simulink model "DeePC_SimulinkV4"  (R2025b)
settings: Solver=FixedStepDiscrete  StartTime=0.0  StopTime=12  FixedStep=0.001  RelTol=1e-3  EnableMultiTasking=on
PreLoadFcn:
  | if ~exist('Ts', 'var')
  | Ts = 0.001;
  | end
  | if ~exist('FPGA_Frequency', 'var')
  | FPGA_Frequency = 75000000;
  | end
  | if ~exist('Tpwm', 'var')
  | Tpwm = 0.005;
  | end
model workspace (MAT data in the model file):
  Sig = Simulink.Signal
  Sig.Dimensions = -1
  Sig.DimensionsMode = 'auto'
  Sig.Complexity = 'auto'
  Sig.SampleTime = -1
  Sig.SamplingMode = 'auto'
  Sig.DataType = 'auto'
values from neighbouring files (symbols this model uses):
  f_pre_r = makeParam(DataStruct.f)    [ExperimentControlCenter_V3.m]
  H = makeParam(DataStruct.H)    [ExperimentControlCenter_V3.m]
  H_p = makeParam(DataStruct.H_p)    [ExperimentControlCenter_V3.m]
  IOscale = makeParam(DataStruct.IOscale)    [ExperimentControlCenter_V3.m]
  l = makeParam(l_val)    [ExperimentControlCenter_V3.m]
  lambda_g = makeParam(lambda_g_list(1))    [ExperimentControlCenter_V3.m]
  lambda_y = 5e2    (= 500)    [ExperimentControlCenter_V3.m]
  N = makeParam(DataStruct.N)    [ExperimentControlCenter_V3.m]
  T_ini = makeParam(DataStruct.T_ini)    [ExperimentControlCenter_V3.m]
  T_switch = makeParam(T_switch_val)    [ExperimentControlCenter_V3.m]
  Ts_ctrl_sl = makeParam(Ts_ctrl)    [ExperimentControlCenter_V3.m]
  U_f = makeParam(DataStruct.U_f)    [ExperimentControlCenter_V3.m]
  Y_f = makeParam(DataStruct.Y_f)    [ExperimentControlCenter_V3.m]
undefined symbols (not defined in the file or in its folder): DiscIntNeverNeededParam, IO397, Pull, pull, up
libraries: simulink x6, speedgoatlib_fpga_analog_io x3, speedgoatlib_fpga_quadrature x3, speedgoatlib_fpga_dio x1, speedgoatlib_fpga_inta x1, speedgoatlib_interrupt x1, speedgoatlib_fpga_pwm x1, speedgoatlib_fpga x1
settings Model: SimulationMode=external  ExtModeEnableFloating=off  Creator=jeffrey.gruenig  LastModifiedBy=gertv
settings SolverCC: ConcurrentTasks=on  PositivePriorityOrder=on  AutoInsertRateTranBlk=on
settings DataIOCC: SaveFormat=StructureWithTime  SaveOutput=off  SaveTime=off
settings OptimizationCC: BlockReduction=off  DefaultParameterBehavior=Inlined  OptimizeBlockIOStorage=off  EnhancedBackFolding=on  PassReuseOutputArgsThreshold=0.0  OptimizeBlockOrder=speed  DifferentSizesBufferReuse=on
settings DebuggingCC: UnderspecifiedInitializationDetection=Classic  MergeDetectMultiDrivingBlocksExec=none  TasksWithSamePriorityMsg=none  ParameterTunabilityLossMsg=error  AllowSymbolicDim=off
settings HardwareCC: ProdBitPerLong=64.0  ProdLongLongMode=on  ProdHWDeviceType=Intel->x86-64 (Linux 64)
settings ModelReferenceCC: PropagateSignalLabelsOutOfModel=off
settings RTWCC: SystemTargetFile=speedgoat.tlc  TLCOptions=-p0  TemplateMakefile=slrealtime_default_tmf  GenerateReport=on  RTWVerbose=off  Toolchain=Simulink Real-Time Toolchain  LaunchReport=on  CodeExecutionProfiling=on  TargetLang=C++  Description=Speedgoat Real-Time Target Machine
settings CodeAppCC: ForceParamTrailComments=on  OperatorAnnotations=on
settings SimulinkRealTimeTargetCC: SLRTFileLogMaxRuns=1.0  ExtModeMaxTrigDuration=10.0  ExtModeStaticAllocSize=1000000.0  ExtModeTransport=0.0  MultiwordLength=2048.0  DynamicStringBufferSize=256.0  PreserveMATLABNamespacesInGeneratedCode=on  SubcomponentCodeInterfacePackaging=Reusable function  InstructionSetFMA=off  LogToMDFFile=off

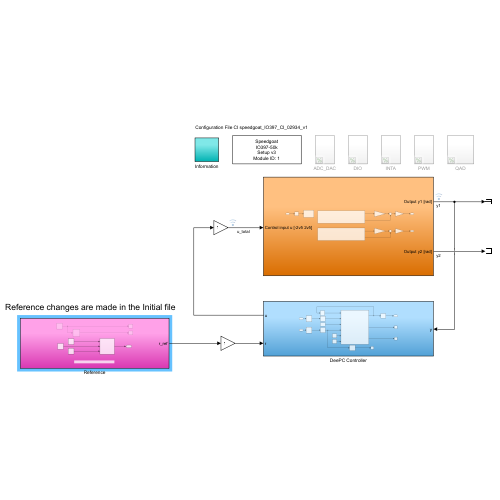
[thumbnail: Simulink's stored preview of the top-level diagram]
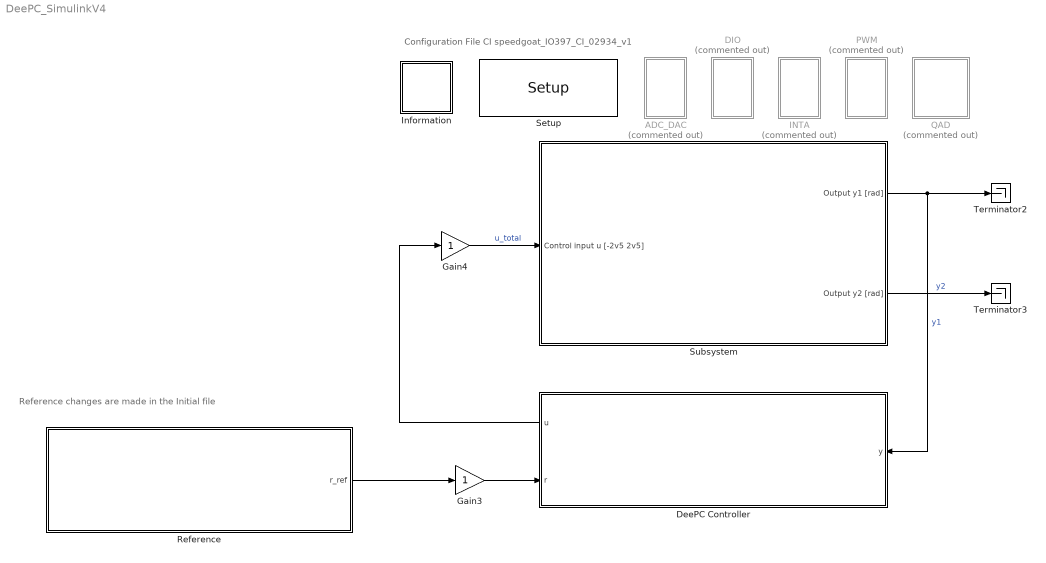
== system DeePC_SimulinkV4 ==
  note: Reference changes are made in the Initial file
  note: Configuration File CI speedgoat_IO397_CI_02934_v1
  ADC_DAC : Subsystem  Commented=on
  DIO : Subsystem  Commented=on
  DeePC Controller : Subsystem
      settings: PortSchema="{\"entries\":[{\"content\":{\"sides\":[{\"content\":{\"connectorIds\":[\"In1\"]},\"type\":\"ConnectorPlacement.EquallySpacedRectSide\",\"uuid\":\"2e71bc44-88de-4f6b-852e-26b86c3fb698\"},{\"content\":{\"connectorIds\":[\"Out1\",\"In2\"],\"side\":\"RIGHT\"},\"type\":\"ConnectorPlacement.EquallySpacedRectSide\",\"uuid\":\"c8a8557f-0bf5-47f4-bae2-a177ab114f93\"},{\"content\":{\"side\":\"TOP\"},\"type\":\"ConnectorPlacement.EquallySpacedRectSide\",\"uuid\":\"9add04b7-c795-4733-b5be-0ba9d1775d75\"},{\"content\":{\"side\":\"BOTTOM\"},\"type\":\"ConnectorPlacement.EquallySpacedRectSide\",\"uuid\":\"f8ea6dec-d938-4893-9b5d-ff6cf4332b98\"}]},\"type\":\"ConnectorPlacement.EquallySpacedConnector\",\"uuid\":\"ed5613c3-599d-4249-97c1-c6090c1efcc5\"}],\"packageUris\":[\"http://schema.mathworks.com/mf0/Connector/R2020b\"],\"version\":\"1.0\"}"
  Gain3 : Gain
  Gain4 : Gain
  INTA : Subsystem  Commented=on
  Information : Subsystem
  PWM : Subsystem  Commented=on
  QAD : Subsystem  Commented=on
  Reference : Subsystem
  Setup : speedgoatlib_fpga/Setup/Setup  board=IO397-50k  id=1  pciSlot=-1  device_id=1  bitstreamFilePath=C:\Users\gertv\Documents\Werk\Continuing Thesis\Matlab\GithubFolder\Section 9 - Experimental Results\ExperimentSet_up\DeePC_Exp  bitstreamFile=speedgoat_IO397_CI_02934_v1.mat  fpgaFreq=75000000  enableDma=off  rearEnb_1=off  rearIO_1=None  rearEnb_2=off  rearIO_2=None  ProgSpiFlash=off  ProgBPIFlash=off  useFpgaDmaController=off  dmaStopOnOverload=on  dmaModeSequential=on  dmaModeParallel=off  dmaTrigFixTime=on  dmaTrigA2B=off  dmaTriggerSourceSel=0  PullRPort15=pull-up 3.3V  PullRPort31=pull-up 3.3V  PullRPort47=pull-up 3.3V  PullRPort63=pull-up 3.3V  diffLineTermination_1=on  diffLineTermination_2=on  diffLineTermination_3=on  diffLineTermination_4=on  diffLineTermination_5=on  diffLineTermination_6=on  diffLineTermination_7=on  diffLineTermination_8=on  diffLineTermination_9=on  diffLineTermination_10=on  diffLineTermination_11=on  diffLineTermination_12=on  diffLineTermination_13=on  diffLineTermination_14=on  diffLineTermination_15=on  diffLineTermination_16=on  diffLineTermination_17=on  diffLineTermination_18=on  diffLineTermination_19=on  diffLineTermination_20=on  diffLineTermination_21=on  diffLineTermination_22=on  diffLineTermination_23=on  diffLineTermination_24=on  diffLineTermination_25=on  diffLineTermination_26=on  diffLineTermination_27=on  diffLineTermination_28=on  diffLineTermination_29=on  diffLineTermination_30=on  diffLineTermination_31=on  diffLineTermination_32=on  ioVoltageDropDown1=3.3V  pullResistorDropDown1_1=Pull-up  pullResistorDropDown1_2=Pull-up  pullResistorDropDown1_3=Pull-up  pullResistorDropDown1_4=Pull-up  pullResistorDropDown1_5=Pull-up  pullResistorDropDown1_6=Pull-up  pullResistorDropDown1_7=Pull-up  pullResistorDropDown1_8=Pull-up  ttlIsImplementedCheckBox1=off  pullResistorDropDown2=Pull-up  ioVoltageDropDown2=3.3V  ttlIsImplementedCheckBox2=off  pullResistorDropDown3=Pull-up  ioVoltageDropDown3=3.3V  ttlIsImplementedCheckBox3=off  pullResistorDropDown4=Pull-up  ioVoltageDropDown4=3.3V  ttlIsImplementedCheckBox4=off  pullResistorDropDown5=Pull-up  ioVoltageDropDown5=3.3V  ttlIsImplementedCheckBox5=off  pullResistorDropDown6=Pull-up  ioVoltageDropDown6=3.3V  ttlIsImplementedCheckBox6=off  pullResistorDropDown7=Pull-up  ioVoltageDropDown7=3.3V  ttlIsImplementedCheckBox7=off  pullResistorDropDown8=Pull-up  ioVoltageDropDown8=3.3V  ttlIsImplementedCheckBox8=off  terminationCheckBox1=off  terminationCheckBox2=off  terminationCheckBox3=off  terminationCheckBox4=off  diffIsImplementedCheckBox1=off  terminationCheckBox5=off  terminationCheckBox6=off  terminationCheckBox7=off  terminationCheckBox8=off  diffIsImplementedCheckBox2=off  terminationCheckBox9=off  terminationCheckBox10=off  terminationCheckBox11=off  terminationCheckBox12=off  diffIsImplementedCheckBox3=off  terminationCheckBox13=off  terminationCheckBox14=off  terminationCheckBox15=off  terminationCheckBox16=off  diffIsImplementedCheckBox4=off  terminationCheckBox17=off  terminationCheckBox18=off  terminationCheckBox19=off  terminationCheckBox20=off  diffIsImplementedCheckBox5=off  terminationCheckBox21=off  terminationCheckBox22=off  terminationCheckBox23=off  terminationCheckBox24=off  diffIsImplementedCheckBox6=off  terminationCheckBox25=off  terminationCheckBox26=off  terminationCheckBox27=off  terminationCheckBox28=off  diffIsImplementedCheckBox7=off  terminationCheckBox29=off  terminationCheckBox30=off  terminationCheckBox31=off  terminationCheckBox32=off  diffIsImplementedCheckBox8=off  PullRPort0_1=pull-up  VioPort0_1=3.3V  PullRPort1_1=pull-up  VioPort1_1=3.3V  PullRPort2_1=pull-up  VioPort2_1=3.3V  PullRPort3_1=pull-up  VioPort3_1=3.3V  PullRPort4_1=pull-up  VioPort4_1=3.3V  PullRPort5_1=pull-up  VioPort5_1=3.3V  PullRPort6_1=pull-up  VioPort6_1=3.3V  diffLineTermination_rear1_1=on  diffLineTermination_rear1_2=on  diffLineTermination_rear1_3=on  diffLineTermination_rear1_4=on  diffLineTermination_rear1_5=on  diffLineTermination_rear1_6=on  diffLineTermination_rear1_7=on  diffLineTermination_rear1_8=on  PullRPort0_2=pull-up  VioPort0_2=3.3V  PullRPort1_2=pull-up  VioPort1_2=3.3V  PullRPort2_2=pull-up  VioPort2_2=3.3V  PullRPort3_2=pull-up  VioPort3_2=3.3V  PullRPort4_2=pull-up  VioPort4_2=3.3V  PullRPort5_2=pull-up  VioPort5_2=3.3V  PullRPort6_2=pull-up  VioPort6_2=3.3V  diffLineTermination_rear2_1=on  diffLineTermination_rear2_2=on  diffLineTermination_rear2_3=on  diffLineTermination_rear2_4=on  diffLineTermination_rear2_5=on  diffLineTermination_rear2_6=on  diffLineTermination_rear2_7=on  diffLineTermination_rear2_8=on
      settings: SourceProductName=IO3xx
  Subsystem : Subsystem
  Terminator2 : Terminator
  Terminator3 : Terminator
  wires:
  Gain4/1 -> Subsystem/1(Control input u [-2v5 2v5])  "u_total"
  Gain3/1 -> DeePC Controller/2(r)
  Subsystem/2(Output y2 [rad]) -> Terminator3/1  "y2"
  Subsystem/1(Output y1 [rad]) -> DeePC Controller/1(y), Terminator2/1  "y1"
  Reference/1(r_ref) -> Gain3/1
  DeePC Controller/1(u) -> Gain4/1

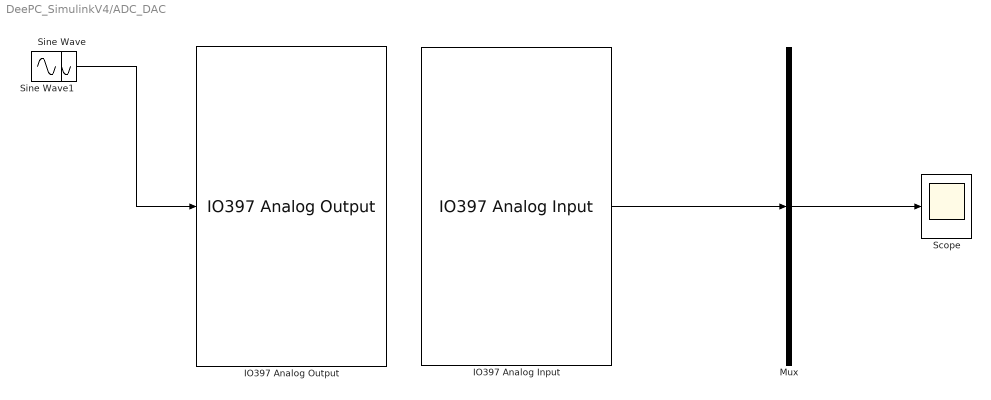
== system DeePC_SimulinkV4/ADC_DAC ==
  IO397 Analog Input : speedgoatlib_fpga_analog_io/IO397/IO397 Analog Input  openMaskCallback=0  id=1  chan=1,  range=+5.12 V  parAiTriggerMode=I/O Module Clock  parAiInternalSignal=None  parAiDioTriggerChannel=1  parAiSampleRate=0  trigger=Initiator  ts=Ts*0.1
      settings: SourceProductName=Analog IO
  IO397 Analog Output : speedgoatlib_fpga_analog_io/IO397/IO397 Analog Output  id=1  chan=1,  initVal=0  resetVal=0  ts=0.001  span=+-10 V
      settings: SourceProductName=Analog IO
  Mux : Mux  Inputs=1
  Scope : Scope
  Sine Wave : Sin  Frequency=2*pi*(1/Ts)/50  SampleTime=Ts
  Sine Wave1 : Sin  Frequency=2*pi*(1/Ts)/50  SampleTime=Ts
  wires:
  Mux/1 -> Scope/1
  IO397 Analog Input/1 -> Mux/1
  Sine Wave/1 -> IO397 Analog Output/1

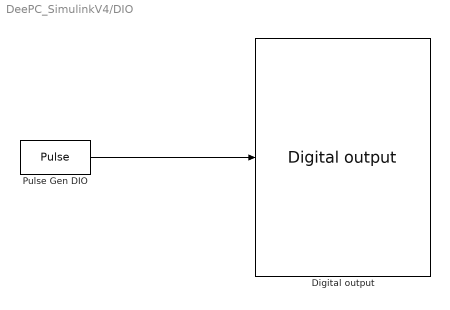
== system DeePC_SimulinkV4/DIO ==
  Digital output : speedgoatlib_fpga_dio/Digital output  id=1  chan=[11:13]  init=[0]  reset=[0]  ts=Ts  vectorizeInput=on
      settings: SourceProductName=Digital
  Pulse Gen DIO : DiscretePulseGenerator  Period=20  PulseWidth=10  PhaseDelay=[0:5:10]  SampleTime=Ts  VectorParams1D=off
  wires:
  Pulse Gen DIO/1 -> Digital output/1

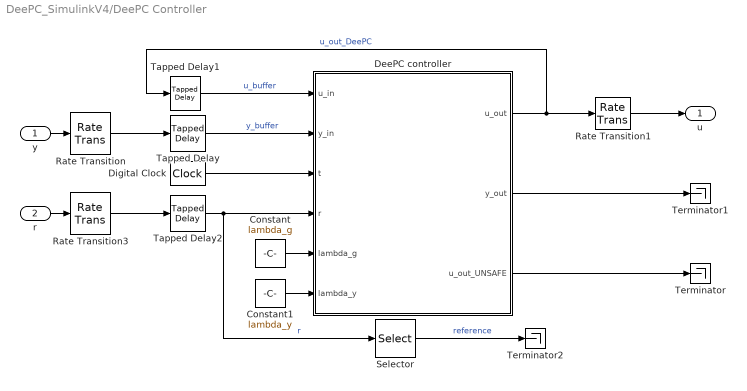
== system DeePC_SimulinkV4/DeePC Controller ==
  y : Inport  PortDimensions=1
  r : Inport  Port=2
  Constant : Constant  Value=lambda_g
  Constant1 : Constant  Value=lambda_y
  DeePC controller : MATLAB Function  TreatAsAtomicUnit=on
  Digital Clock : DigitalClock  SampleTime=Ts_ctrl_sl
  Rate Transition : RateTransition  OutPortSampleTime=Ts_ctrl_sl
  Rate Transition1 : RateTransition  Deterministic=off  OutPortSampleTime=1e-3
  Rate Transition3 : RateTransition  OutPortSampleTime=Ts_ctrl_sl
  Selector : Selector  InputPortWidth=l  IndexOptions=Index vector (dialog)  Indices=[l]  OutputSizes=1
  Tapped Delay : simulink/Discrete/Tapped Delay  vinit=0.0  samptime=-1  NumDelays=l  DelayOrder=Oldest  includeCurrent=off
  Tapped Delay1 : simulink/Discrete/Tapped Delay  vinit=0.0  samptime=-1  NumDelays=l  DelayOrder=Oldest  includeCurrent=off
  Tapped Delay2 : simulink/Discrete/Tapped Delay  vinit=0.0  samptime=-1  NumDelays=l  DelayOrder=Oldest  includeCurrent=off
  Terminator : Terminator
  Terminator1 : Terminator
  Terminator2 : Terminator
  u : Outport
  wires:
  Tapped Delay/1 -> DeePC controller/2(y_in)  "y_buffer"
  Tapped Delay1/1 -> DeePC controller/1(u_in)  "u_buffer"
  Constant/1 -> DeePC controller/5(lambda_g)
  Digital Clock/1 -> DeePC controller/3(t)
  y/1 -> Rate Transition/1
  Rate Transition/1 -> Tapped Delay/1
  Constant1/1 -> DeePC controller/6(lambda_y)
  DeePC controller/1(u_out) -> Tapped Delay1/1, Rate Transition1/1  "u_out_DeePC"
  r/1 -> Rate Transition3/1
  Tapped Delay2/1 -> DeePC controller/4(r), Selector/1  "r"
  Rate Transition3/1 -> Tapped Delay2/1
  Rate Transition1/1 -> u/1
  DeePC controller/3(u_out_UNSAFE) -> Terminator/1
  DeePC controller/2(y_out) -> Terminator1/1
  Selector/1 -> Terminator2/1  "reference"

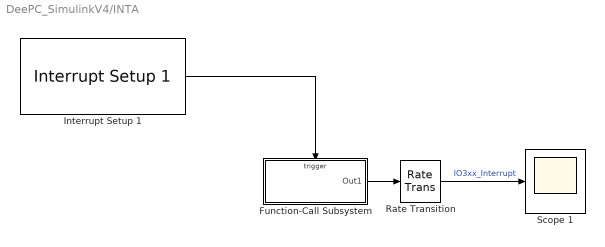
== system DeePC_SimulinkV4/INTA ==
  Function-Call Subsystem : Subsystem  TreatAsAtomicUnit=on
  Interrupt Setup 1 : speedgoatlib_interrupt/Interrupt Setup 1  parModuleTrigger=off  parPollingMode=off  parPriorityConf=High  parPriority=241  confStartFcn=''  confStopFcn=''  confIsrFcn=''  confMapFcn=''  confHookFile=''  confIrqNr='-1'  confIsPolling=off  confModID='1'  confSelectedInt=Speedgoat IO397-50k interrupt  confSelectedId=1  confSelectedChannel=[]  confData=[]
  Rate Transition : RateTransition  Integrity=off
  "Scope 1 " : Scope
  wires:
  Rate Transition/1 -> "Scope 1 "/1  "IO3xx_Interrupt"
  Function-Call Subsystem/1(Out1) -> Rate Transition/1
  Interrupt Setup 1/1 -> Function-Call Subsystem/Trigger

== system DeePC_SimulinkV4/Information ==
  note: Front I/O (Analog):
      | From Pin To Pin Tested Functionality
      | 9 1 / 2 DAC channel 1 to ADC channel 1
      | Front I/O:
      | From Pin To Pin Tested Functionality
      | 3b 12b PWM - A channel 1 to INTA channel 1
      | 13b 6b DIO channel 11 to QAD - A channel 1
      | 14b 7b DIO channel 12 to QAD - B channel 1
      | 15b 8b DIO channel 13 to QAD - C_Index channel 1

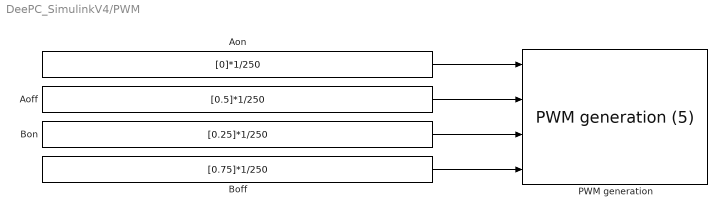
== system DeePC_SimulinkV4/PWM ==
  Aoff : Constant  Value=[0.5]*1/250  OutDataTypeStr=Inherit: Inherit via back propagation  SampleTime=-1
  Aon : Constant  Value=[0]*1/250  VectorParams1D=off  OutDataTypeStr=Inherit: Inherit via back propagation  SampleTime=-1
  Boff : Constant  Value=[0.75]*1/250  OutDataTypeStr=Inherit: Inherit via back propagation  SampleTime=-1
  Bon : Constant  Value=[0.25]*1/250  OutDataTypeStr=Inherit: Inherit via back propagation  SampleTime=-1
  PWM generation : speedgoatlib_fpga_pwm/PWM generation (5)  id=1  chan=[1]  board=Please select...  ts=0.001  enableDma=off  pciSlot=-1  delay=0  symmetric=Asymmetric - On and Off are freely configurable  b_is_complement_of_a=Independent of PWM A output  deadband=[0.0]  period=[1/250]  frequency=250  ticks=299999  a_on=0  a_off=0.5e-3  pwm_a_dc=[0.0]  b_on=0.25e-3  b_off=0.75e-3  pwm_b_dc=[0]  c_on=[0.0]  c_off=[0.0]  protection=Disabled: A and B can be high at the same moment  enable_latch_half_period=off  pwm_update=At period starts  bit_width_pwm_gen=24  trigger_duration=[100e-6]  trigger_period_start=on  trigger_half_of_the_period=off  trigger_a_on=off  trigger_a_off=off  trigger_b_on=off  trigger_b_off=off  show_a_input=on  show_b_input=on  show_c_input=off  show_period_input=off  show_force_stop_input=off  idle_a=Low when PWM generation is halted  idle_b=Low when PWM generation is halted  idle_c=Low when PWM generation is halted  cancels_pwm_generation=on  invert_a=off  invert_b=off  invert_c=off
      settings: SourceProductName=PWM
  wires:
  Boff/1 -> PWM generation/4
  Bon/1 -> PWM generation/3
  Aoff/1 -> PWM generation/2
  Aon/1 -> PWM generation/1

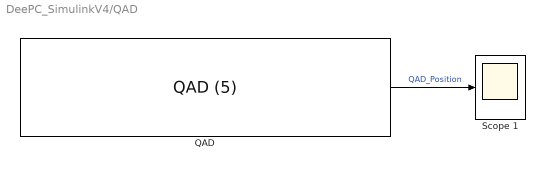
== system DeePC_SimulinkV4/QAD ==
  QAD : speedgoatlib_fpga_quadrature/QAD (5)  id=1  chan=[1]  sampleTime=0.001  enableDma=on  numOfSlots=[16]  sensorType=Capture A + B Signal  interpolatePosition=off  swapAB=off  indexControlMode=Ignore Index  latchMode=Disabled  gateIndex=No Gating  speedFilterWidth=4  showInputSpeedFilterWidth=off  glitchFilterSeconds=106.7e-9  glitchFilterSecondsEff=106.7e-9  showInputClearPosition=off  showInputClearIndexFound=off  showOutputPosition=on  showOutputTurn=off  showOutputSpeed=off  showOutputIndexFound=off  showOutputLastPulse=off
      settings: SourceProductName=Quadrature
  "Scope 1 " : Scope
  wires:
  QAD/1 -> "Scope 1 "/1  "QAD_Position"

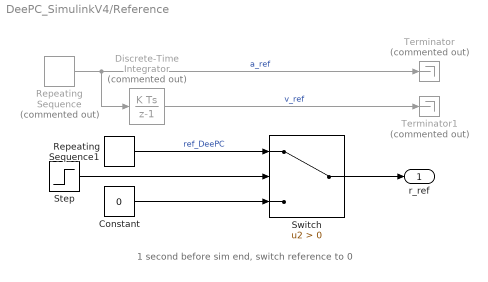
== system DeePC_SimulinkV4/Reference ==
  note: 1 second before sim end, switch reference to 0
  Constant : Constant  Value=0
  Discrete-Time Integrator : DiscreteIntegrator  Commented=on  SampleTime=-1  ICPrevOutput=DiscIntNeverNeededParam  ICPrevScaledInput=DiscIntNeverNeededParam
  Repeating Sequence : simulink/Sources/Repeating Sequence  Commented=on  rep_seq_t=t_tab  rep_seq_y=a_tab
  Repeating Sequence1 : simulink/Sources/Repeating Sequence  rep_seq_t=t_tab  rep_seq_y=p_tab
  Step : Step  Time=10  Before=1  After=0  SampleTime=0
  Switch : Switch  Criteria=u2 > Threshold  SaturateOnIntegerOverflow=off  InputSameDT=off
  Terminator : Terminator  Commented=on
  Terminator1 : Terminator  Commented=on
  r_ref : Outport
  wires:
  Repeating Sequence1/1 -> Switch/1  "ref_DeePC"
  Discrete-Time Integrator/1 -> Terminator1/1  "v_ref"
  Repeating Sequence/1 -> Discrete-Time Integrator/1, Terminator/1  "a_ref"
  Switch/1 -> r_ref/1
  Constant/1 -> Switch/3
  Step/1 -> Switch/2

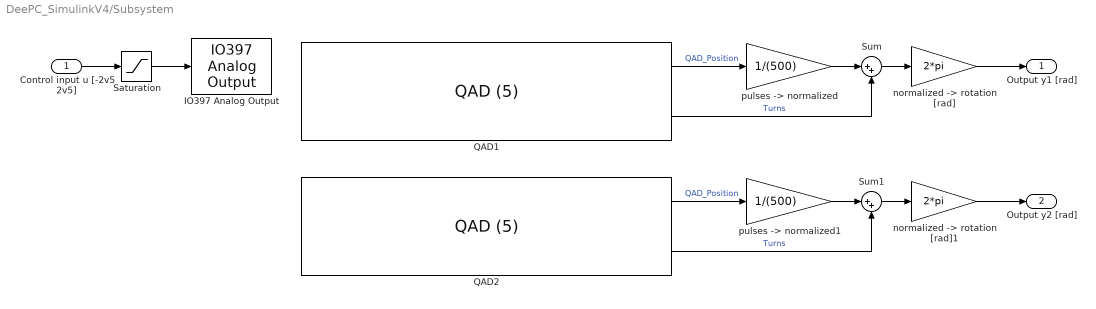
== system DeePC_SimulinkV4/Subsystem ==
  Control input u [-2v5 2v5] : Inport
  IO397 Analog Output : speedgoatlib_fpga_analog_io/IO397/IO397 Analog Output  id=1  chan=1,  initVal=0  resetVal=1  ts=0.001  span=+-5 V
      settings: SourceProductName=Analog IO
  QAD1 : speedgoatlib_fpga_quadrature/QAD (5)  id=1  chan=[1]  sampleTime=0.001  numOfSlots=500  sensorType=Capture A + B Signal  interpolatePosition=off  swapAB=off  indexControlMode=Ignore Index  latchMode=Disabled  gateIndex=No Gating  speedFilterWidth=1  showInputSpeedFilterWidth=off  glitchFilterSeconds=0  glitchFilterSecondsEff=0  showInputClearPosition=off  showInputClearIndexFound=off  showOutputPosition=on  showOutputTurn=on  showOutputSpeed=off  showOutputIndexFound=off  showOutputLastPulse=off
      settings: SourceProductName=Quadrature
  QAD2 : speedgoatlib_fpga_quadrature/QAD (5)  id=1  chan=[2]  sampleTime=0.001  numOfSlots=500  sensorType=Capture A + B Signal  interpolatePosition=off  swapAB=off  indexControlMode=Ignore Index  latchMode=Disabled  gateIndex=No Gating  speedFilterWidth=1  showInputSpeedFilterWidth=off  glitchFilterSeconds=0  glitchFilterSecondsEff=0  showInputClearPosition=off  showInputClearIndexFound=off  showOutputPosition=on  showOutputTurn=on  showOutputSpeed=off  showOutputIndexFound=off  showOutputLastPulse=off
      settings: SourceProductName=Quadrature
  Saturation : Saturate  UpperLimit=2.5  LowerLimit=-2.5
  Sum : Sum  Inputs=|++
  Sum1 : Sum  Inputs=|++
  "normalized -> rotation [rad]" : Gain  Gain=2*pi
  "normalized -> rotation [rad]1" : Gain  Gain=2*pi
  "pulses -> normalized" : Gain  Gain=1/(500)
  "pulses -> normalized1" : Gain  Gain=1/(500)
  Output y1 [rad] : Outport
  Output y2 [rad] : Outport  Port=2
  wires:
  Saturation/1 -> IO397 Analog Output/1
  Sum/1 -> "normalized -> rotation [rad]"/1
  "normalized -> rotation [rad]"/1 -> Output y1 [rad]/1
  QAD1/1 -> "pulses -> normalized"/1  "QAD_Position"
  QAD1/2 -> Sum/2  "Turns"
  "pulses -> normalized"/1 -> Sum/1
  Control input u [-2v5 2v5]/1 -> Saturation/1
  "pulses -> normalized1"/1 -> Sum1/1
  QAD2/2 -> Sum1/2  "Turns"
  QAD2/1 -> "pulses -> normalized1"/1  "QAD_Position"
  Sum1/1 -> "normalized -> rotation [rad]1"/1
  "normalized -> rotation [rad]1"/1 -> Output y2 [rad]/1

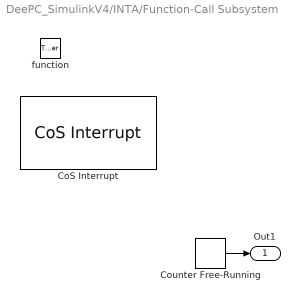
== system DeePC_SimulinkV4/INTA/Function-Call Subsystem ==
  function : TriggerPort  TriggerType=function-call  VariantControl=Variant
  CoS Interrupt : speedgoatlib_fpga_inta/CoS Interrupt  id=1  ts=-1  debounce=0  delay=0  polarity=1
      settings: SourceProductName=Interrupt
  Counter Free-Running : simulink/Sources/Counter Free-Running  NumBits=32  tsamp=-1
  Out1 : Outport  InitialOutput=[0]  VectorParamsAs1DForOutWhenUnconnected=off
  wires:
  Counter Free-Running/1 -> Out1/1

== matlab function DeePC_SimulinkV4/DeePC Controller/DeePC controller ==
  settings: updateMethod=DISCRETE  sampleTime=Ts_ctrl_sl
  data: u_in input; y_in input; u_out output; t input; y_out output; r input; lambda_g input; lambda_y input; Ts_ctrl_sl parameter; T_switch parameter; f_pre_r parameter; u_out_UNSAFE output; H_p parameter; U_f parameter; Y_f parameter; H parameter; T_ini parameter; N parameter; IOscale parameter
function [u_out, y_out, u_out_UNSAFE] = DeePCNoShift(u_in, y_in, t, r, lambda_g, lambda_y, Ts_ctrl_sl, T_switch, f_pre_r, H_p, U_f, Y_f, H, T_ini, N, IOscale)
% The DeePC controller employs an online optimization based on data from a
% "data-gathering" step. 

% Extract the data properties from H = createMatrices()
    % f_pre_r = DataStruct.f;
    % H_p = DataStruct.H_p;
    % U_f = DataStruct.U_f;
    % Y_f = DataStruct.Y_f;
    % Ts = DataStruct.Ts; %Absolute sampling time
    % H = DataStruct.H;
    % T_ini = DataStruct.T_ini;
    % N = DataStruct.N;
    % IOscale = DataStruct.IOscale;
    % u_bounds = DataStruct.u_bounds;
    % y_bounds = DataStruct.y_bounds;
    u_bounds = 0; y_bounds = 0;
    scale_u = IOscale(1); scale_y = IOscale(2);

    persistent slack_size
    if isempty(slack_size)
    slack_size = round(T_ini/Ts_ctrl_sl);
    end

   persistent g_prev
    if isempty(g_prev)
        if isempty(lambda_y) || lambda_y == 0
            g_prev = zeros(size(H,1),1);
        else
            g_prev = zeros(size(H,1)+slack_size,1);
         end
    end
    
    persistent opts
    if isempty(opts)
        opts = optimoptions('quadprog', 'Display', 'off', 'ConstraintTolerance', 1e-7,'OptimalityTolerance',1e-7,'MaxIterations',1500,'Algorithm','active-set');
    end
    u_out_UNSAFE = 0; %allocate a special variable to check predicted suggested inputs

    if t <= T_switch
        % Before DeePC is triggered
        u_out = 0;
        y_out = 0;
    else
        g_initial = g_prev;
        if mod(t, Ts_ctrl_sl) ~= 0
            u_out = u_in(end);
            y_out = 0;
            return
        end
        
        % Constructing r matrix
        r_mat = r./scale_y;
        f = f_pre_r'*r_mat;
        
        
        y_ini = y_in;
        u_ini = u_in;

        l_ini = [u_ini; y_ini];
        W = 2*(H + lambda_g * eye(size(H)));

        % OPTIONAL: ADD SAFETY CONSTRAINTS
        n = length(f);
        A_ineq = zeros(0,n);
        b_ineq = zeros(0,1);
        if ~all(u_bounds == 0)
            A_ineq = [-U_f; U_f];
            b_ineq = repmat([-u_bounds(1); u_bounds(2)], round(N/Ts_ctrl_sl), 1);
        end
        
        if ~all(y_bounds == 0)
            A_ineq = [A_ineq; -Y_f; Y_f]; 
            b_ineq = [b_ineq; repmat([-y_bounds(1); y_bounds(2)], round(N/Ts_ctrl_sl),1)];
        end

        if isempty(lambda_y) || lambda_y == 0
            % Start regular optimalization
            [g, ~, exitflag] = quadprog(W, f, A_ineq, b_ineq, H_p, l_ini, [], [], g_initial, opts);
            % [g_slack, ~, exitflag] = quadprog(W_slack, f_slack, A_ineq_slack, b_ineq, H_slack, l_ini, [], [], [], options);
            g_prev = g;

        else
            % QP with slack variable
            slack_var_mat = eye(round(T_ini/Ts_ctrl_sl)).*lambda_y;
            W_slack = blkdiag(W,slack_var_mat);
           
            H_p_slack = [H_p, [zeros(size(H_p,1) - round(T_ini/Ts_ctrl_sl), round(T_ini/Ts_ctrl_sl)); eye(round(T_ini/Ts_ctrl_sl))]];
            f_slack = [f; zeros(size(slack_var_mat,1),1)]; 
            A_ineq_slack = [A_ineq, zeros(size(A_ineq,1),size(slack_var_mat,1))];
            
            [g_slack, ~, exitflag] = quadprog(W_slack, f_slack, A_ineq_slack, b_ineq, H_p_slack, l_ini, [], [], g_initial, opts);

            % [g_slack,exitflag] = mpcActiveSetSolver(W_slack,f_slack,A_ineq_slack, b_ineq, H_slack,l_ini, IA0, options);
            g = g_slack(1:end-slack_size); % Extract g
            g_prev = [g;zeros(slack_size,1)];
        end

        %Safety measure 1: if no feasible solution is gathered, turn of
        %controller
        if exitflag ~= 1
             warning('DeePC infeasible at time t=%.3f. Holding last input.', t);
            u_out = u_in(end);
            y_out = y_in(end);
            
            if isempty(lambda_y) || lambda_y == 0
                g_prev = zeros(size(H,1),1);
            else
                g_prev = zeros(size(H,1)+slack_size,1);
            end
        else
    
        % Predict control input and output
        u_predicted = U_f * g;
        y_predicted = Y_f * g;  

        % rescale our outputs and inputs
        u_predicted = u_predicted.*scale_u ;
        y_predicted = y_predicted.*scale_y ;

        % Take the first sample
        u_out = u_predicted(1);
        y_out = y_predicted(1);
        u_out_UNSAFE = u_out; %allocate a special variable to check predicted suggested inputs

        %Safety measure 2: if computed inputs exceed the safe limit, turn
        %off controller
        if any(abs(u_predicted(1))> 1.5) 
            warning('predicted inputs too large. The controller is shut off for safety')
            u_out = 0;
        end
        end
    end
end
